simulink model "ADCS_sim"  (R2018b)
settings: Solver=VariableStepAuto  StartTime=0.0  StopTime=T
values from neighbouring files (symbols this model uses):
  A_i = [A_sc(1); A_sc(2); A_sc(3); A_sc(1); A_sc(2); A_sc(3);            A_sa; A_sa; A_sa; A_sa]'    [data_setup.m]
  G = [1 10 1e-4 1e-4 1e-4 1e-4]    [main.m]
  mag_res = [1; 1; 1]*1e-3    [data_setup.m]
  n = length(t)    [main.m]
  n_i = [eye(3), -eye(3), n_sa, -n_sa, n_sa, -n_sa]    [data_setup.m]
  P = zeros(18,18,nF)    [main_test_ekf.m]
  r_i = [CG_1, CG_2, CG_3, CG_4, CG_5, CG_6, CG_7, CG_8, CG_9, CG_10]    [data_setup.m]
  rhoD = ones(1,10)*0.1    [data_setup.m]
  rhoS = [ones(1,6)*0.5, ones(1,4)*0.8]    [data_setup.m]
undefined symbols (not defined in the file or in its folder): A, a, alp_w, Ar, Ar_star, B, C, e, epsilon, fov_star, fov_sun, g1_0, H0, in, Ir, Ixyz, L, mi, n_star_sens, n_sun, n_sun_sens, omega0, omegaE, R_e, R_sun, RAAN, rate_mag, rate_star, rate_sun, sig_mag, sig_star, sig_sun, star_cat, th0
libraries: simulink_extras x9, vrlib x6, dspmathops x5, simulink x5, sharedutil x2, dspmtrx3 x1, dspfactors x1
(part 1 of 2)
settings Model: Creator=Francesco  LastModifiedBy=Francesco
settings DebuggingCC: UnderSpecifiedDimensionMsg=warning

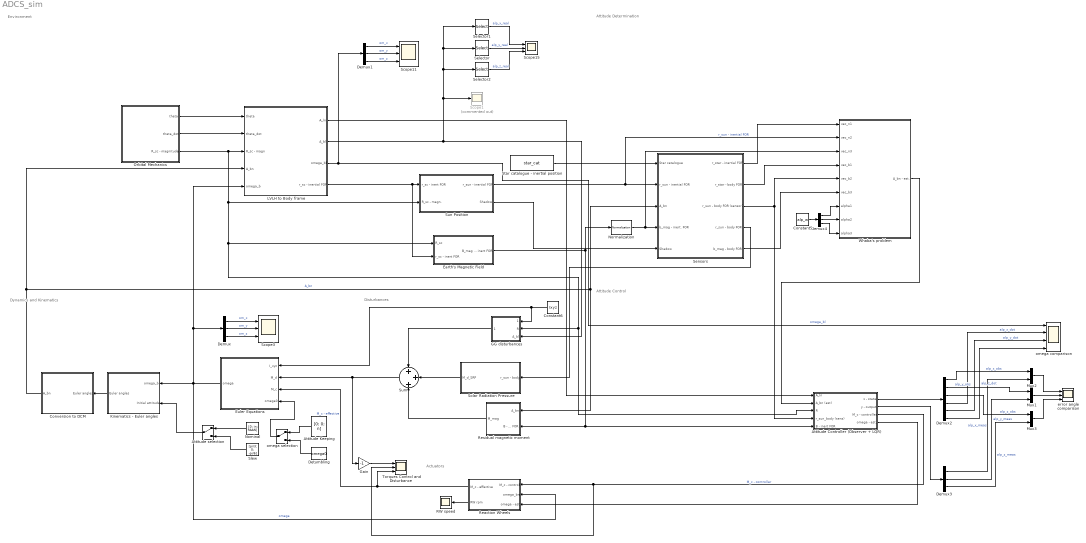
== system ADCS_sim ==
  note: Attitude Control
  note: Dynamics and Kinematics
  note: Attitude Determination
  note: Environment
  note: Actuators
  note: Disturbances
  Attitude Controller (Observer + LQR) : Subsystem
  Attitude Keeping : Constant  Value=[0; 0; n]  VectorParams1D=off
  Attitude selection : ManualSwitch
  Constant5 : Constant  Value=alp_w
  Constant6 : Constant  Value=Ixyz
  Conversion to DCM : Subsystem
  Demux{,1,3..4} (4 alike) : Demux  Outputs=3
  Demux2 : Demux  Outputs=6
  Detumbling : Constant  Value=omega0
  Earth's Magnetic Field : Subsystem
  Euler Equations : Subsystem
  GG disturbances : Subsystem
  Gain : Gain  Gain=-1
  Kinematics - Euler angles : Subsystem
  LVLH to Body frame : Subsystem
  Mux1 : Mux  Inputs=2
  Mux2 : Mux  Inputs=2
  Mux3 : Mux  Inputs=2
  Nominal : Constant  Value=[0; in; RAAN]
  Normalization : dspmathops/Normalization  NormType=2-norm  Bias=1e-10  NormOver=Each column  Dimension=1  roundingMode=Floor  overflowMode=off  accumDataTypeStr=Inherit: Same as product output  accumLastDataTypeStr=Inherit: Same as product output  outputDataTypeStr=Inherit: Same as product output  outputMin=[]  outputMax=[]  outputLastDataTypeStr=Inherit: Same as product output
      settings: SourceProductName=DSP System Toolbox
  Orbital Mechanics : Subsystem
  RW speed : Scope
  Reaction Wheels : Subsystem
  Residual magnetic moment : Subsystem
  Scope1 : Scope  Commented=on
  Scope11 : Scope  NumInputPorts=3
  Scope15 : Scope  NumInputPorts=3
  Scope3 : Scope  NumInputPorts=3
  Selector : Selector  NumberOfDimensions=2  InputPortWidth=3  IndexOptions=Index vector (dialog),Index vector (dialog)  Indices=3,1  OutputSizes=1,1
  Selector1 : Selector  NumberOfDimensions=2  InputPortWidth=3  IndexOptions=Index vector (dialog),Index vector (dialog)  Indices=2,3  OutputSizes=1,1
  Selector2 : Selector  NumberOfDimensions=2  InputPortWidth=3  IndexOptions=Index vector (dialog),Index vector (dialog)  Indices=1,2  OutputSizes=1,1
  Sensors : Subsystem
  Slew : Constant  Value=[pi/3; 0; -pi/6]
  Solar Radiation Pressure : Subsystem  TreatAsAtomicUnit=on
  Star catalogue - inertial position : Constant  Value=star_cat
  Sum : Sum  Inputs=+++
  Sun Position : Subsystem
  Torques Control and Disturbance : Scope  NumInputPorts=3
  Whaba's problem : Subsystem
  error angle comparison : Scope  NumInputPorts=3
  omega comparison : Scope  NumInputPorts=4
  omega selection : ManualSwitch
  wires:
  Demux/2 -> Scope3/2  "om_y"
  LVLH to Body frame/2(A_bl) -> GG disturbances/3(A_bl), Selector/1, Selector1/1, Selector2/1, Scope1/1
  Demux/1 -> Scope3/1  "om_x"
  Demux1/2 -> Scope11/2  "om_y"
  LVLH to Body frame/3(omega_bl) -> omega comparison/1, Demux1/1  "omega_bl"
  Sun Position/1(r_sun - inertial FOR) -> Sensors/2(r_sun - inertial FOR), Whaba's problem/2(vec_n2)  "r_sun - inertial FOR"
  Demux1/1 -> Scope11/1  "om_x"
  Demux/3 -> Scope3/3  "om_z"
  Demux1/3 -> Scope11/3  "om_z"
  Orbital Mechanics/1(theta) -> LVLH to Body frame/1(theta)
  Orbital Mechanics/2(theta_dot) -> LVLH to Body frame/2(theta_dot)
  Euler Equations/1(omega) -> Demux/1, LVLH to Body frame/5(omega_b), Kinematics - Euler angles/1(omega_b), Reaction Wheels/2(omega_bn)  "omega"
  Attitude Keeping/1 -> omega selection/1
  Constant6/1 -> GG disturbances/1("Ix, Iy, Iz"), Euler Equations/1(I_xyz)
  Conversion to DCM/1(A_bn) -> Sensors/3(A_bn), Residual magnetic moment/1(A_bn), LVLH to Body frame/4(A_bn)  "A_bn"
  Residual magnetic moment/1(M_mag) -> Sum/3
  Solar Radiation Pressure/1(M_d_SRP) -> Sum/2
  GG disturbances/1(M_d_GG) -> Sum/1
  Orbital Mechanics/3(R_sc - magnitude) -> LVLH to Body frame/3(R_sc - magn), Attitude Controller (Observer + LQR)/3(R), GG disturbances/2(R), Earth's Magnetic Field/1(R_sc), Sun Position/2(R_sc - magn.)
  LVLH to Body frame/4(r_sc - inertial FOR) -> Earth's Magnetic Field/2(r_sc - inert FOR), Sun Position/1(r_sc - inert FOR)
  Sensors/4(r_sun - body FOR) -> Solar Radiation Pressure/1(r_sun - body)
  Demux2/1 -> Mux2/1  "alp_x_obs"
  Demux2/2 -> Mux1/1  "alp_y_obs"
  Demux3/1 -> Mux2/2  "alp_x_meas"
  Demux3/2 -> Mux1/2  "alp_y_meas"
  Demux2/4 -> omega comparison/2  "alp_x_dot"
  Demux2/5 -> omega comparison/3  "alp_y_dot"
  Demux2/3 -> Mux3/1  "alp_z_obs"
  Demux3/3 -> Mux3/2  "alp_z_meas"
  Demux2/6 -> omega comparison/4  "alp_z_dot"
  Sum/1 -> Euler Equations/2(M_d), Gain/1
  Gain/1 -> Torques Control and Disturbance/1
  Reaction Wheels/1(M_c - effective) -> Euler Equations/3(M_c), Torques Control and Disturbance/3  "M_c - effective"
  Kinematics - Euler angles/1(Euler angles) -> Conversion to DCM/1(Euler angles)
  Star catalogue - inertial position/1 -> Sensors/1(Star catalogue)
  omega selection/1 -> Euler Equations/4(omega0)
  Nominal/1 -> Attitude selection/1
  Attitude selection/1 -> Kinematics - Euler angles/2(Initial attitude)
  Earth's Magnetic Field/1(B_mag - inert FOR) -> Normalization/1, Residual magnetic moment/2(B - inert FOR), Attitude Controller (Observer + LQR)/5(B - inert FOR)
  Constant5/1 -> Demux4/1
  Demux4/1 -> Whaba's problem/7(alpha1)
  Demux4/2 -> Whaba's problem/8(alpha2)
  Demux4/3 -> Whaba's problem/9(alpha3)
  Detumbling/1 -> omega selection/2
  Sun Position/2(Shadow) -> Sensors/5(Shadow)
  Normalization/1 -> Whaba's problem/3(vec_n3), Sensors/4(b_mag - inert. FOR)
  Sensors/5(b_mag - body FOR) -> Whaba's problem/6(vec_b3)
  Sensors/3(r_sun - body FOR (sensor)) -> Attitude Controller (Observer + LQR)/4(r_sun_body (sens)), Whaba's problem/5(vec_b2)
  Sensors/2(r_star - body FOR) -> Whaba's problem/4(vec_b1)
  Selector/1 -> Scope15/2  "alp_y_real"
  Selector1/1 -> Scope15/1  "alp_x_real"
  Selector2/1 -> Scope15/3  "alp_z_real"
  Sensors/1(r_star - inertial FOR) -> Whaba's problem/1(vec_n1)
  Mux2/1 -> error angle comparison/1
  Mux1/1 -> error angle comparison/2
  Mux3/1 -> error angle comparison/3
  Slew/1 -> Attitude selection/2
  Reaction Wheels/2(RW rpm) -> RW speed/1
  Attitude Controller (Observer + LQR)/2(y - output) -> Demux3/1
  Attitude Controller (Observer + LQR)/1(x - state) -> Demux2/1
  Attitude Controller (Observer + LQR)/3(M_c - controller) -> Torques Control and Disturbance/2, Reaction Wheels/1(M_c - control)  "M_c - controller"
  LVLH to Body frame/1(A_ln) -> Attitude Controller (Observer + LQR)/1(A_ln)
  Whaba's problem/1(A_bn - est.) -> Attitude Controller (Observer + LQR)/2(A_bn (est))
  Attitude Controller (Observer + LQR)/4(omega - est.) -> Reaction Wheels/3(omega - est)

== system ADCS_sim/Attitude Controller (Observer + LQR) ==
  A_ln : Inport
  A_bn (est) : Inport  Port=2
  R : Inport  Port=3
  r_sun_body (sens) : Inport  Port=4
  B - inert FOR : Inport  Port=5
  Disturbance Estimator : Subsystem
  "Observer and Controller " : Subsystem
  x - state : Outport
  y - output : Outport  Port=2
  M_c - controller : Outport  Port=3
  omega - est. : Outport  Port=4
  wires:
  "Observer and Controller "/3(M_c - controller) -> M_c - controller/1
  Disturbance Estimator/1(M_d - est.) -> "Observer and Controller "/3(M_d)
  A_ln/1 -> "Observer and Controller "/1(A_ln), Disturbance Estimator/2(A_ln)
  B - inert FOR/1 -> Disturbance Estimator/5(B - inert FOR)
  A_bn (est)/1 -> Disturbance Estimator/4(A_bn), "Observer and Controller "/2(A_bn - est)
  r_sun_body (sens)/1 -> Disturbance Estimator/3(r_sun_body)
  "Observer and Controller "/2(y - output) -> y - output/1
  "Observer and Controller "/1(x - state) -> x - state/1
  "Observer and Controller "/4(omega - est.) -> omega - est./1
  R/1 -> Disturbance Estimator/1(R)

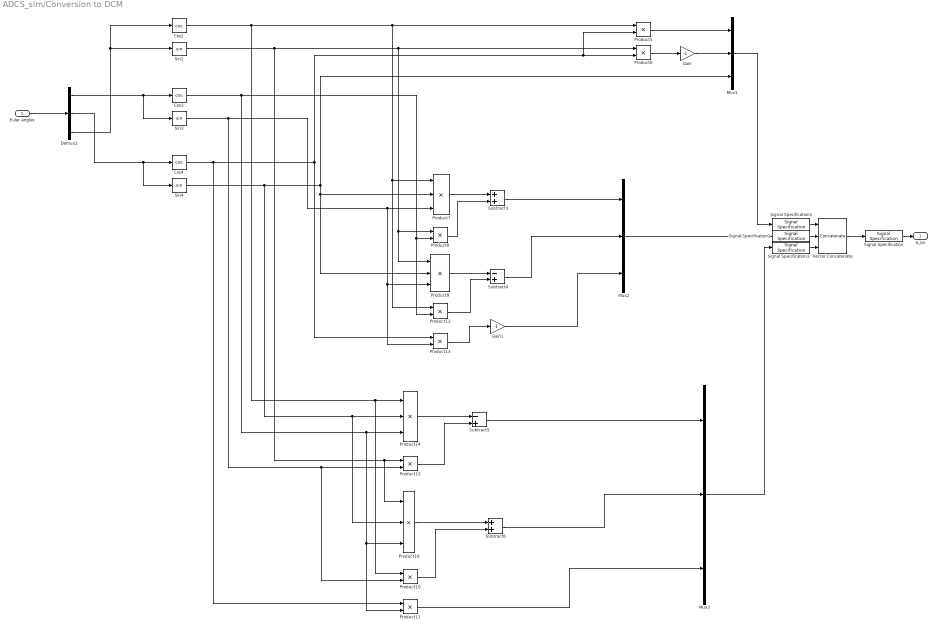
== system ADCS_sim/Conversion to DCM ==
  Euler angles : Inport
  Cos2 : Trigonometry  Operator=cos
  Cos3 : Trigonometry  Operator=cos
  Cos4 : Trigonometry  Operator=cos
  Demux2 : Demux  Outputs=3
  Gain : Gain  Gain=-1
  Gain1 : Gain  Gain=-1
  Mux1 : Mux  Inputs=3
  Mux2 : Mux  Inputs=3
  Mux3 : Mux  Inputs=3
  Product{5..6,8,10..13,15} (8 alike) : Product
  Product{7,9,14,16} (4 alike) : Product  Inputs=3
  Signal Specification : SignalSpecification  Dimensions=[3;3]
  Signal Specification1 : SignalSpecification  Dimensions=[3;1]
  Signal Specification2 : SignalSpecification  Dimensions=[3;1]
  Signal Specification3 : SignalSpecification  Dimensions=[3;1]
  Sin2 : Trigonometry
  Sin3 : Trigonometry
  Sin4 : Trigonometry
  Subtract3 : Sum
  Subtract4 : Sum  Inputs=-+
  Subtract5 : Sum  Inputs=-+
  Subtract6 : Sum
  Vector Concatenate : Concatenate  NumInputs=3  Mode=Multidimensional array  ConcatenateDimension=2
  A_bn : Outport
  wires:
  Product5/1 -> Mux1/1
  Euler angles/1 -> Demux2/1
  Cos2/1 -> Product12/1, Product7/1, Product5/1, Product10/1, Product14/1
  Demux2/3 -> Sin2/1, Cos2/1
  Cos4/1 -> Product11/1, Product13/1, Product5/2, Product6/2
  Subtract5/1 -> Mux3/1
  Mux2/1 -> Signal Specification2/1
  Product15/1 -> Subtract5/2
  Product10/1 -> Subtract6/2
  Sin3/1 -> Product10/2, Product15/2, Product13/2, Product9/3, Product7/3
  Sin2/1 -> Product16/1, Product15/1, Product9/1, Product8/1, Product6/1
  Mux1/1 -> Signal Specification1/1
  Sin4/1 -> Product9/2, Product7/2, Mux1/3, Product16/2, Product14/2
  Product13/1 -> Gain1/1
  Demux2/2 -> Cos4/1, Sin4/1
  Product6/1 -> Gain/1
  Product8/1 -> Subtract3/2
  Product11/1 -> Mux3/3
  Product12/1 -> Subtract4/2
  Demux2/1 -> Sin3/1, Cos3/1
  Cos3/1 -> Product12/2, Product8/2, Product11/2, Product16/3, Product14/3
  Gain1/1 -> Mux2/3
  Product9/1 -> Subtract4/1
  Gain/1 -> Mux1/2
  Subtract3/1 -> Mux2/1
  Subtract6/1 -> Mux3/2
  Product16/1 -> Subtract6/1
  Product14/1 -> Subtract5/1
  Product7/1 -> Subtract3/1
  Subtract4/1 -> Mux2/2
  Vector Concatenate/1 -> Signal Specification/1
  Mux3/1 -> Signal Specification3/1
  Signal Specification/1 -> A_bn/1
  Signal Specification1/1 -> Vector Concatenate/1
  Signal Specification2/1 -> Vector Concatenate/2
  Signal Specification3/1 -> Vector Concatenate/3

== system ADCS_sim/Earth's Magnetic Field ==
  R_sc : Inport
  r_sc - inert FOR : Inport  Port=2
  Constant6 : Constant  Value=H0
  Constant7 : Constant  Value=R_e
  Constant8 : Constant  Value=3
  Divide1 : Product  Inputs=*/
  Dot Product : DotProduct  InputSameDT=on  OutDataTypeStr=Inherit: Inherit via internal rule
  Gain : Gain  Gain=3
  Power : Math  Operator=pow  SaturateOnIntegerOverflow=on
  Product : Product
  Product1 : Product
  Product2 : Product
  Subsystem1 : Subsystem
  Subtract : Sum  Inputs=+-
  B_mag - inert FOR : Outport
  wires:
  Constant7/1 -> Divide1/1
  Power/1 -> Product/2
  Gain/1 -> Product1/2
  Constant6/1 -> Product/1
  r_sc - inert FOR/1 -> Product1/1, Dot Product/1
  Dot Product/1 -> Gain/1
  R_sc/1 -> Divide1/2
  Product/1 -> Product2/1
  Product1/1 -> Subtract/1
  Product2/1 -> B_mag - inert FOR/1
  Subtract/1 -> Product2/2
  Constant8/1 -> Power/2
  Divide1/1 -> Power/1
  Subsystem1/1("m_hat - inert FOR ") -> Dot Product/2, Subtract/2

== system ADCS_sim/Euler Equations ==
  I_xyz : Inport
  M_d : Inport  Port=2
  M_c : Inport  Port=3
  omega0 : Inport  Port=4
  Demux : Demux  Outputs=3
  Demux1 : Demux  Outputs=3
  Divide : Product  Inputs=/*
  Integrator : Integrator  InitialConditionSource=external  InitialCondition=[0.45; 0.52; 0.55]
  Mux : Mux  Inputs=3
  Product : Product  Inputs=3
  Product1 : Product  Inputs=3
  Product2 : Product  Inputs=3
  Subtract : Sum  Inputs=+-
  Subtract1 : Sum  Inputs=+-
  Subtract2 : Sum  Inputs=+-
  Sum : Sum  Inputs=|++
  Sum1 : Sum  Inputs=|++
  omega : Outport
  wires:
  Divide/1 -> Integrator/1  "omega_dot"
  Demux1/1 -> Product2/3, Product1/2
  Demux1/3 -> Product1/3, Product/2
  Subtract1/1 -> Product1/1
  Integrator/1 -> omega/1, Demux1/1  "omega"
  Demux1/2 -> Product2/2, Product/3
  Subtract/1 -> Product/1
  Demux/2 -> Subtract2/2, Subtract/1
  Demux/1 -> Subtract2/1, Subtract1/2
  Demux/3 -> Subtract/2, Subtract1/1
  Mux/1 -> Sum1/1
  omega0/1 -> Integrator/2
  Product1/1 -> Mux/2
  Product/1 -> Mux/1
  Product2/1 -> Mux/3
  Sum/1 -> Sum1/2
  I_xyz/1 -> Divide/1, Demux/1
  Subtract2/1 -> Product2/1
  M_c/1 -> Sum/1
  M_d/1 -> Sum/2
  Sum1/1 -> Divide/2

== system ADCS_sim/GG disturbances ==
  "Ix, Iy, Iz" : Inport
  R : Inport  Port=2
  A_bl : Inport  Port=3
  Constant : Constant  Value=[1; 0; 0]
  Constant1 : Constant  Value=3
  Constant2 : Constant  Value=mi
  Demux2 : Demux  Outputs=3
  Demux3 : Demux  Outputs=3
  Divide : Product  Inputs=*/
  Gain : Gain  Gain=3
  Matrix Multiply2 : Product  Multiplication=Matrix(*)
  Mux : Mux  Inputs=3
  Power : Math  Operator=pow  SaturateOnIntegerOverflow=on
  Product1 : Product  Inputs=4
  Product2 : Product  Inputs=4
  Product3 : Product  Inputs=4
  Subtract1 : Sum  Inputs=+-
  Subtract2 : Sum  Inputs=+-
  Subtract3 : Sum  Inputs=+-
  M_d_GG : Outport
  wires:
  Mux/1 -> M_d_GG/1
  Product2/1 -> Mux/2
  Product3/1 -> Mux/3
  Product1/1 -> Mux/1
  Matrix Multiply2/1 -> Demux3/1
  Subtract3/1 -> Product3/2
  Subtract1/1 -> Product1/2
  Subtract2/1 -> Product2/2
  Demux3/1 -> Product3/3, Product2/3
  "Ix, Iy, Iz"/1 -> Demux2/1
  Demux3/2 -> Product3/4, Product1/4
  Demux2/3 -> Subtract2/2, Subtract1/1
  Constant/1 -> Matrix Multiply2/2
  Demux2/2 -> Subtract3/1, Subtract1/2
  Demux3/3 -> Product2/4, Product1/3
  Demux2/1 -> Subtract3/2, Subtract2/1
  Gain/1 -> Product3/1, Product2/1, Product1/1
  A_bl/1 -> Matrix Multiply2/1
  R/1 -> Power/1
  Constant1/1 -> Power/2
  Divide/1 -> Gain/1
  Power/1 -> Divide/2
  Constant2/1 -> Divide/1

== system ADCS_sim/Kinematics - Euler angles ==
  omega_b : Inport
  Initial attitude : Inport  Port=2
  Cos : Trigonometry  Operator=cos
  Cos1 : Trigonometry  Operator=cos
  Demux : Demux  Outputs=3
  Demux1 : Demux  Outputs=3
  Divide : Product  Inputs=/*
  Integrator : Integrator  InitialConditionSource=external  InitialCondition=[pi/2; pi/2; 0]
  Mux : Mux  Inputs=3
  Product{,1..4} (5 alike) : Product
  Sin : Trigonometry
  Sin1 : Trigonometry
  Subtract : Sum  Inputs=+-
  Subtract1 : Sum
  Subtract2 : Sum  Inputs=-+
  Terminator : Terminator
  Euler angles : Outport
  wires:
  omega_b/1 -> Demux/1
  Demux1/1 -> Terminator/1  "phi"
  Demux1/2 -> Sin/1, Cos/1  "theta"
  Demux1/3 -> Sin1/1, Cos1/1  "psi"
  Demux/1 -> Product3/2, Product/2  "om_u"
  Cos1/1 -> Product2/1, Product/1
  Demux/2 -> Product2/2, Product1/2  "om_v"
  Sin1/1 -> Product3/1, Product1/1
  Product/1 -> Subtract/1
  Product1/1 -> Subtract/2
  Subtract/1 -> Divide/2
  Cos/1 -> Divide/1
  Divide/1 -> Product4/2, Mux/1
  Product2/1 -> Subtract1/1
  Product3/1 -> Subtract1/2
  Subtract1/1 -> Mux/2
  Mux/1 -> Integrator/1  "E.A. dot"
  Demux/3 -> Subtract2/2  "om_w"
  Subtract2/1 -> Mux/3
  Product4/1 -> Subtract2/1
  Sin/1 -> Product4/1
  Integrator/1 -> Demux1/1, Euler angles/1
  Initial attitude/1 -> Integrator/2

== system ADCS_sim/LVLH to Body frame ==
  theta : Inport
  theta_dot : Inport  Port=2
  R_sc - magn : Inport  Port=3
  A_bn : Inport  Port=4
  omega_b : Inport  Port=5
  Constant4 : Constant  Value=in
  Constant7 : Constant  Value=RAAN
  Position vector calculator : Subsystem
  Subsystem1 : Subsystem
  inert2lvlh : Subsystem
  A_ln : Outport
  A_bl : Outport  Port=2
  omega_bl : Outport  Port=3
  r_sc - inertial FOR : Outport  Port=4
  wires:
  Constant4/1 -> inert2lvlh/2(i)
  inert2lvlh/1(A_ln) -> Subsystem1/3(A_ln), A_ln/1  "A_ln"
  theta_dot/1 -> Subsystem1/1(theta_dot)
  Subsystem1/1(A_bl) -> A_bl/1  "A_bl"
  omega_b/1 -> Subsystem1/4(omega_b)
  theta/1 -> Position vector calculator/1(theta), inert2lvlh/1(theta)
  A_bn/1 -> Subsystem1/2(A_bn)
  Subsystem1/2(omega_bl) -> omega_bl/1
  Constant7/1 -> inert2lvlh/3(RAAN)
  Position vector calculator/1(r_n) -> r_sc - inertial FOR/1  "r_sc - inertial FOR"
  inert2lvlh/2(PF 2 ECI) -> Position vector calculator/3(PF 2 ECI)
  R_sc - magn/1 -> Position vector calculator/2(R)

== system ADCS_sim/Orbital Mechanics ==
  Constant : Constant  Value=th0
  Constant1 : Constant  Value=a
  Constant2 : Constant  Value=e
  Constant3 : Constant  Value=mi
  Orbital Mechanics evolut. : Subsystem
  theta : Outport
  theta_dot : Outport  Port=2
  R_sc - magnitude : Outport  Port=3
  wires:
  Constant1/1 -> Orbital Mechanics evolut./2(a)
  Orbital Mechanics evolut./1(theta) -> theta/1
  Orbital Mechanics evolut./3(theta_dot) -> theta_dot/1
  Constant3/1 -> Orbital Mechanics evolut./3(mi)
  Constant2/1 -> Orbital Mechanics evolut./4(e)
  Orbital Mechanics evolut./2(R) -> R_sc - magnitude/1
  Constant/1 -> Orbital Mechanics evolut./1(theta0)

== system ADCS_sim/Reaction Wheels ==
  M_c - control : Inport
  omega_bn : Inport  Port=2
  omega - est : Inport  Port=3
  Reaction Wheels controller : Subsystem
  Reaction Wheels response : Subsystem
  rad/s 2 rpm : Gain  Gain=60/2/pi
  M_c - effective : Outport
  RW rpm : Outport  Port=2
  wires:
  M_c - control/1 -> Reaction Wheels controller/2(M_c - control)
  rad/s 2 rpm/1 -> RW rpm/1  "RW rpm"
  Reaction Wheels controller/1(omega_r) -> rad/s 2 rpm/1, Reaction Wheels response/2(omega_r)
  Reaction Wheels response/1(M_c - effective) -> M_c - effective/1
  omega_bn/1 -> Reaction Wheels response/1(omega_bn)
  omega - est/1 -> Reaction Wheels controller/1(omega_bn)

== system ADCS_sim/Residual magnetic moment ==
  A_bn : Inport
  B - inert FOR : Inport  Port=2
  Constant6 : Constant  Value=mag_res
  Cross Product : vrlib/Utilities/Cross Product
      settings: SourceProductBaseCode=VR
  Matrix Multiply1 : Product  Multiplication=Matrix(*)
  M_mag : Outport
  wires:
  Matrix Multiply1/1 -> Cross Product/2  "b - body FOR"
  B - inert FOR/1 -> Matrix Multiply1/2
  Constant6/1 -> Cross Product/1
  Cross Product/1 -> M_mag/1
  A_bn/1 -> Matrix Multiply1/1

== system ADCS_sim/Sensors ==
  Star catalogue : Inport
  r_sun - inertial FOR : Inport  Port=2
  A_bn : Inport  Port=3
  b_mag - inert. FOR : Inport  Port=4
  Shadow : Inport  Port=5
  Magnetometer error : Subsystem
  Matrix Multiply : Product  Inputs=3  Multiplication=Matrix(*)
  Matrix Multiply1 : Product  Multiplication=Matrix(*)
  Matrix Multiply2 : Product  Multiplication=Matrix(*)
  Product : Product
  Star Sensor error : Subsystem
  Star selector : Subsystem
  Subsystem : Subsystem
  Sun Sensor error : Subsystem
  r_star - inertial FOR : Outport
  r_star - body FOR : Outport  Port=2
  r_sun - body FOR (sensor) : Outport  Port=3
  r_sun - body FOR : Outport  Port=4
  b_mag - body FOR : Outport  Port=5
  wires:
  A_bn/1 -> Matrix Multiply/2, Subsystem/2(A_bn), Star selector/2(A_bn)
  r_sun - inertial FOR/1 -> Product/2
  Star catalogue/1 -> Star selector/1(Star catalogue)
  Star selector/1(r_star - body FOR) -> Matrix Multiply1/2
  Star Sensor error/1(A_eps) -> Matrix Multiply1/1
  Matrix Multiply1/1 -> r_star - body FOR/1
  Star selector/2(r_star - inertial FOR) -> r_star - inertial FOR/1
  Subsystem/1(r_sun - body FOR (sensor)) -> Matrix Multiply2/2
  Sun Sensor error/1(A_eps) -> Matrix Multiply2/1
  Subsystem/2(r_sun -  body FOR) -> r_sun - body FOR/1
  Matrix Multiply2/1 -> r_sun - body FOR (sensor)/1
  b_mag - inert. FOR/1 -> Matrix Multiply/3
  Magnetometer error/1(A_eps) -> Matrix Multiply/1
  Matrix Multiply/1 -> b_mag - body FOR/1
  Shadow/1 -> Product/1
  Product/1 -> Subsystem/1(r_sun - inert FOR)

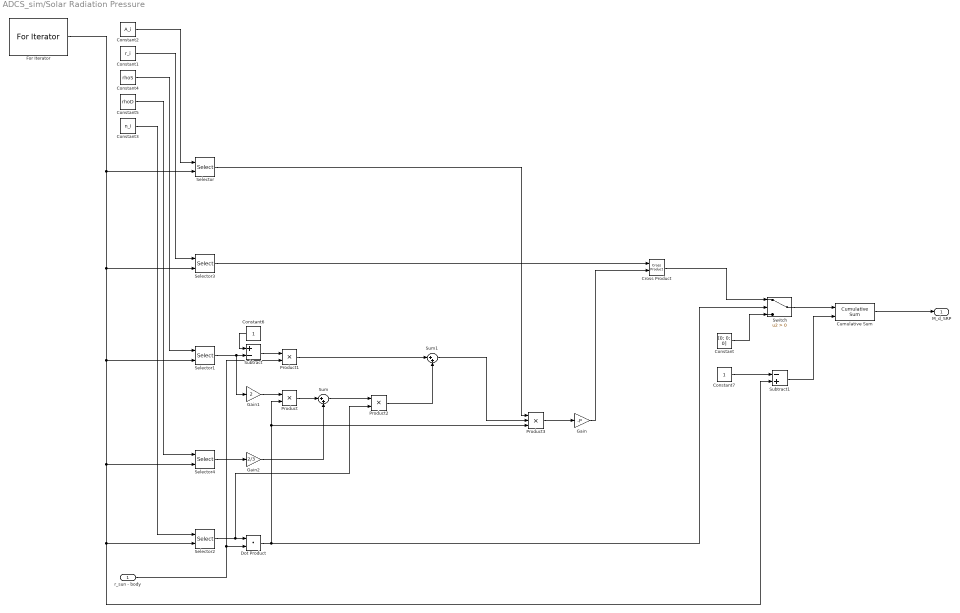
== system ADCS_sim/Solar Radiation Pressure ==
  r_sun - body : Inport
  Constant : Constant  Value=[0; 0; 0]
  Constant1 : Constant  Value=r_i
  Constant2 : Constant  Value=A_i
  Constant3 : Constant  Value=n_i
  Constant4 : Constant  Value=rhoS
  Constant5 : Constant  Value=rhoD
  Constant6 : Constant
  Constant7 : Constant
  Cross Product : vrlib/Utilities/Cross Product
      settings: SourceProductBaseCode=VR
  Cumulative Sum : dspmathops/Cumulative Sum  dim=Channels (running sum)  reset_popup=Falling edge  roundingMode=Floor  overflowMode=off  outputDataTypeStr=Inherit: Same as accumulator  outputMin=[]  outputMax=[]  outputLastDataTypeStr=Inherit: Same as accumulator
      settings: SourceProductName=DSP System Toolbox
  Dot Product : DotProduct  InputSameDT=on  OutDataTypeStr=Inherit: Inherit via internal rule
  For Iterator : ForIterator  IterationLimit=length(A_i)
  Gain : Gain  Gain=-P
  Gain1 : Gain  Gain=2
  Gain2 : Gain  Gain=2/3
  Product : Product
  Product1 : Product
  Product2 : Product
  Product3 : Product  Inputs=3
  Selector{,1..4} (5 alike) : Selector  NumberOfDimensions=2  InputPortWidth=3  IndexOptions=Select all,Index vector (port)  Indices=[1 3],1  OutputSizes=1,1
  Subtract : Sum  Inputs=+-
  Subtract1 : Sum  Inputs=-+
  Sum : Sum  Inputs=|++
  Sum1 : Sum  Inputs=|++
  Switch : Switch  Criteria=u2 > Threshold
  M_d_SRP : Outport
  wires:
  For Iterator/1 -> Selector/2, Selector3/2, Subtract1/2, Selector2/2, Selector4/2, Selector1/2
  Selector/1 -> Product3/1
  Selector3/1 -> Cross Product/1
  Constant3/1 -> Selector2/1
  Selector2/1 -> Product2/2, Dot Product/1
  Constant1/1 -> Selector3/1
  Constant2/1 -> Selector/1
  r_sun - body/1 -> Product1/2, Dot Product/2
  Constant4/1 -> Selector1/1
  Constant5/1 -> Selector4/1
  Selector1/1 -> Subtract/2, Gain1/1
  Constant6/1 -> Subtract/1
  Subtract/1 -> Product1/1
  Dot Product/1 -> Product/2, Product3/3, Switch/2
  Gain1/1 -> Product/1
  Selector4/1 -> Gain2/1
  Product/1 -> Sum/1
  Gain2/1 -> Sum/2
  Sum/1 -> Product2/1
  Product1/1 -> Sum1/1
  Product2/1 -> Sum1/2
  Sum1/1 -> Product3/2
  Product3/1 -> Gain/1
  Gain/1 -> Cross Product/2
  Constant/1 -> Switch/3
  Cross Product/1 -> Switch/1
  Switch/1 -> Cumulative Sum/1
  Subtract1/1 -> Cumulative Sum/2
  Constant7/1 -> Subtract1/1
  Cumulative Sum/1 -> M_d_SRP/1

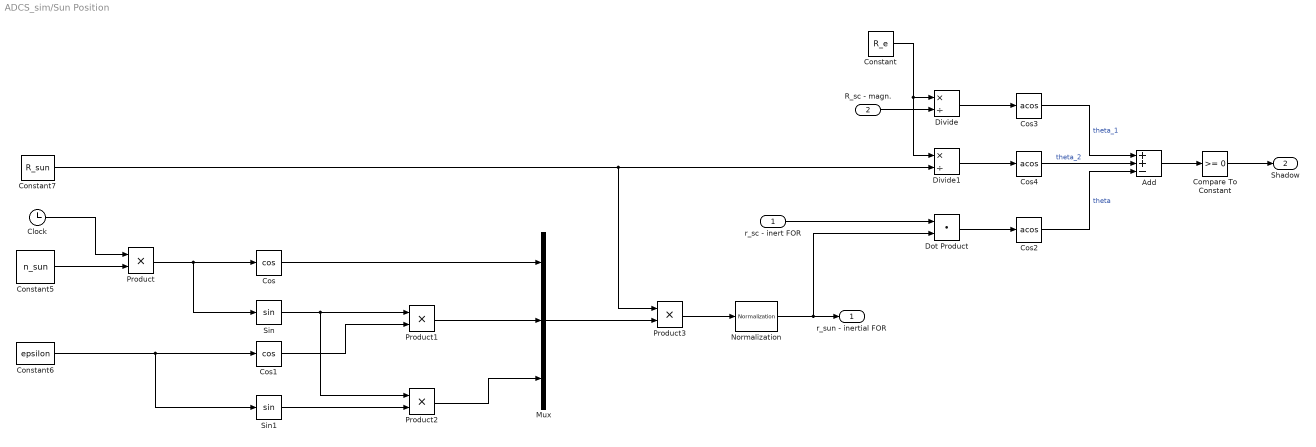
== system ADCS_sim/Sun Position ==
  r_sc - inert FOR : Inport
  R_sc - magn. : Inport  Port=2
  Add : Sum  Inputs=++-
  Clock : Clock
  Compare To Constant : simulink/Logic and Bit Operations/Compare To Constant  relop=>=  const=0  OutDataTypeStr=boolean
  Constant : Constant  Value=R_e
  Constant5 : Constant  Value=n_sun
  Constant6 : Constant  Value=epsilon
  Constant7 : Constant  Value=R_sun
  Cos : Trigonometry  Operator=cos
  Cos1 : Trigonometry  Operator=cos
  Cos2 : Trigonometry  Operator=acos
  Cos3 : Trigonometry  Operator=acos
  Cos4 : Trigonometry  Operator=acos
  Divide : Product  Inputs=*/
  Divide1 : Product  Inputs=*/
  Dot Product : DotProduct  InputSameDT=on  OutDataTypeStr=Inherit: Inherit via internal rule
  Mux : Mux  Inputs=3
  Normalization : dspmathops/Normalization  NormType=2-norm  Bias=1e-10  NormOver=Each column  Dimension=1  roundingMode=Floor  overflowMode=off  accumDataTypeStr=Inherit: Same as product output  accumLastDataTypeStr=Inherit: Same as product output  outputDataTypeStr=Inherit: Same as product output  outputMin=[]  outputMax=[]  outputLastDataTypeStr=Inherit: Same as product output
      settings: SourceProductName=DSP System Toolbox
  Product{,1..3} (4 alike) : Product
  Sin : Trigonometry
  Sin1 : Trigonometry
  r_sun - inertial FOR : Outport
  Shadow : Outport  Port=2
  wires:
  Sin/1 -> Product2/1, Product1/1
  Cos/1 -> Mux/1
  Product/1 -> Sin/1, Cos/1
  Mux/1 -> Product3/2
  Constant6/1 -> Sin1/1, Cos1/1
  Product2/1 -> Mux/3
  Product1/1 -> Mux/2
  Product3/1 -> Normalization/1
  Constant5/1 -> Product/2
  Cos1/1 -> Product1/2
  Clock/1 -> Product/1
  Sin1/1 -> Product2/2
  Constant7/1 -> Product3/1, Divide1/2
  Normalization/1 -> Dot Product/2, r_sun - inertial FOR/1
  r_sc - inert FOR/1 -> Dot Product/1
  Dot Product/1 -> Cos2/1
  Cos2/1 -> Add/3  "theta"
  Constant/1 -> Divide1/1, Divide/1
  R_sc - magn./1 -> Divide/2
  Divide/1 -> Cos3/1
  Divide1/1 -> Cos4/1
  Cos3/1 -> Add/1  "theta_1"
  Cos4/1 -> Add/2  "theta_2"
  Add/1 -> Compare To Constant/1
  Compare To Constant/1 -> Shadow/1

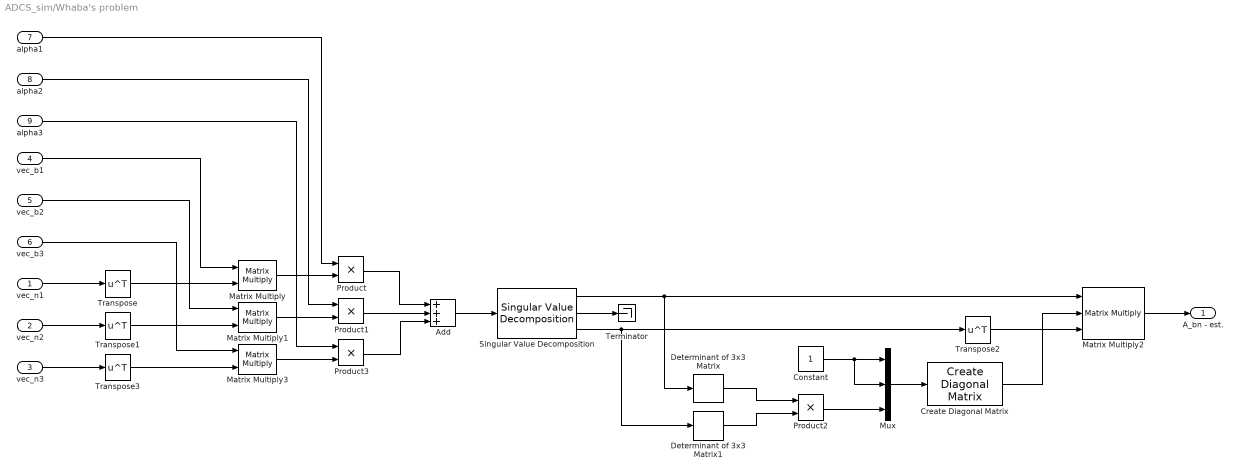
== system ADCS_sim/Whaba's problem ==
  vec_n1 : Inport
  vec_n2 : Inport  Port=2
  vec_n3 : Inport  Port=3
  vec_b1 : Inport  Port=4
  vec_b2 : Inport  Port=5
  vec_b3 : Inport  Port=6
  alpha1 : Inport  Port=7
  alpha2 : Inport  Port=8
  alpha3 : Inport  Port=9
  Add : Sum  Inputs=+++
  Constant : Constant
  Create Diagonal Matrix : dspmtrx3/Create Diagonal Matrix
      settings: SourceProductName=DSP System Toolbox  SourceProductBaseCode=DS
  Determinant of 3x3 Matrix : sharedutil/Determinant of 3x3 Matrix  aMode=aMode
      settings: SourceProductName=Aerospace Blockset  SourceProductBaseCode=AE
  Determinant of 3x3 Matrix1 : sharedutil/Determinant of 3x3 Matrix  aMode=aMode
      settings: SourceProductName=Aerospace Blockset  SourceProductBaseCode=AE
  Matrix Multiply : Product  Multiplication=Matrix(*)
  Matrix Multiply1 : Product  Multiplication=Matrix(*)
  Matrix Multiply2 : Product  Inputs=3  Multiplication=Matrix(*)
  Matrix Multiply3 : Product  Multiplication=Matrix(*)
  Mux : Mux  Inputs=3
  Product{,1..3} (4 alike) : Product
  Singular Value Decomposition : dspfactors/Singular Value Decomposition  wantv=on  wanterr=off  SimulateUsing=Interpreted execution
      settings: SourceProductName=DSP System Toolbox  SourceProductBaseCode=DS
  Terminator : Terminator
  Transpose{,1..3} (4 alike) : Math  Operator=transpose  SaturateOnIntegerOverflow=on
  A_bn - est. : Outport
  wires:
  vec_n1/1 -> Transpose/1
  vec_n2/1 -> Transpose1/1
  Transpose/1 -> Matrix Multiply/2
  vec_b1/1 -> Matrix Multiply/1
  Transpose1/1 -> Matrix Multiply1/2
  vec_b2/1 -> Matrix Multiply1/1
  Matrix Multiply/1 -> Product/2
  Matrix Multiply1/1 -> Product1/2
  alpha2/1 -> Product1/1
  alpha1/1 -> Product/1
  Product/1 -> Add/1
  Product1/1 -> Add/2
  Add/1 -> Singular Value Decomposition/1
  Singular Value Decomposition/2 -> Terminator/1
  Singular Value Decomposition/1 -> Determinant of 3x3 Matrix/1, Matrix Multiply2/1
  Singular Value Decomposition/3 -> Transpose2/1, Determinant of 3x3 Matrix1/1
  Determinant of 3x3 Matrix/1 -> Product2/1
  Determinant of 3x3 Matrix1/1 -> Product2/2
  Product2/1 -> Mux/3
  Constant/1 -> Mux/2, Mux/1
  Mux/1 -> Create Diagonal Matrix/1
  Create Diagonal Matrix/1 -> Matrix Multiply2/2
  Transpose2/1 -> Matrix Multiply2/3
  Matrix Multiply2/1 -> A_bn - est./1
  Product3/1 -> Add/3
  Matrix Multiply3/1 -> Product3/2
  Transpose3/1 -> Matrix Multiply3/2
  vec_n3/1 -> Transpose3/1
  vec_b3/1 -> Matrix Multiply3/1
  alpha3/1 -> Product3/1

== system ADCS_sim/Attitude Controller (Observer + LQR)/Disturbance Estimator ==
  R : Inport
  A_ln : Inport  Port=2
  r_sun_body : Inport  Port=3
  A_bn : Inport  Port=4
  B - inert FOR : Inport  Port=5
  Constant5 : Constant  Value=Ixyz
  GG disturbances1 : Subsystem
  Matrix Multiply2 : Product  Multiplication=Matrix(*)
  Solar Radiation Pressure : Subsystem  TreatAsAtomicUnit=on
  Subsystem3 : Subsystem
  Sum1 : Sum  Inputs=+++
  Transpose : Math  Operator=transpose  SaturateOnIntegerOverflow=on
  M_d - est. : Outport
  wires:
  GG disturbances1/1(M_d_GG) -> Sum1/1
  Constant5/1 -> GG disturbances1/1("Ix, Iy, Iz")
  Subsystem3/1(M_mag) -> Sum1/3
  Solar Radiation Pressure/1(M_d_SRP) -> Sum1/2
  Sum1/1 -> M_d - est./1
  r_sun_body/1 -> Solar Radiation Pressure/1(r_sun - body)
  R/1 -> GG disturbances1/2(R)
  B - inert FOR/1 -> Subsystem3/2(B - inert FOR)
  A_ln/1 -> Transpose/1
  Transpose/1 -> Matrix Multiply2/2
  A_bn/1 -> Subsystem3/1(A_bn), Matrix Multiply2/1
  Matrix Multiply2/1 -> GG disturbances1/3(A_bl)

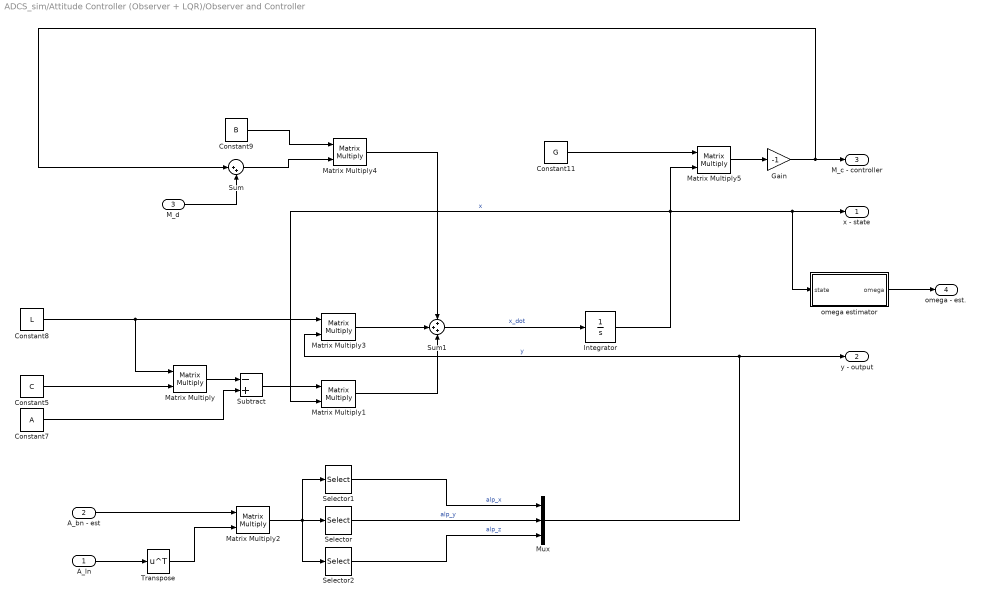
== system ADCS_sim/Attitude Controller (Observer + LQR)/Observer and Controller  ==
  A_ln : Inport
  A_bn - est : Inport  Port=2
  M_d : Inport  Port=3
  Constant11 : Constant  Value=G
  Constant5 : Constant  Value=C
  Constant7 : Constant  Value=A
  Constant8 : Constant  Value=L
  Constant9 : Constant  Value=B
  Gain : Gain  Gain=-1
  Integrator : Integrator  InitialCondition=[0; 0; 0; 0; 0; 0]
  Matrix Multiply{,1..5} (6 alike) : Product  Multiplication=Matrix(*)
  Mux : Mux  Inputs=3
  Selector : Selector  NumberOfDimensions=2  InputPortWidth=3  IndexOptions=Index vector (dialog),Index vector (dialog)  Indices=3,1  OutputSizes=1,1
  Selector1 : Selector  NumberOfDimensions=2  InputPortWidth=3  IndexOptions=Index vector (dialog),Index vector (dialog)  Indices=2,3  OutputSizes=1,1
  Selector2 : Selector  NumberOfDimensions=2  InputPortWidth=3  IndexOptions=Index vector (dialog),Index vector (dialog)  Indices=1,2  OutputSizes=1,1
  Subtract : Sum  Inputs=-+
  Sum : Sum  Inputs=|++
  Sum1 : Sum  Inputs=+++
  Transpose : Math  Operator=transpose  SaturateOnIntegerOverflow=on
  omega estimator : Subsystem
  x - state : Outport
  y - output : Outport  Port=2
  M_c - controller : Outport  Port=3
  omega - est. : Outport  Port=4
  wires:
  Matrix Multiply4/1 -> Sum1/1
  Matrix Multiply2/1 -> Selector2/1, Selector1/1, Selector/1
  Constant9/1 -> Matrix Multiply4/1
  Integrator/1 -> Matrix Multiply1/2, Matrix Multiply5/2, omega estimator/1(state), x - state/1  "x"
  Matrix Multiply5/1 -> Gain/1
  Selector2/1 -> Mux/3  "alp_z"
  Matrix Multiply3/1 -> Sum1/2
  Selector1/1 -> Mux/1  "alp_x"
  Constant5/1 -> Matrix Multiply/2
  Mux/1 -> y - output/1, Matrix Multiply3/2  "y"
  Constant8/1 -> Matrix Multiply/1, Matrix Multiply3/1
  Selector/1 -> Mux/2  "alp_y"
  Matrix Multiply/1 -> Subtract/1
  Matrix Multiply1/1 -> Sum1/3
  Transpose/1 -> Matrix Multiply2/2
  Subtract/1 -> Matrix Multiply1/1
  A_ln/1 -> Transpose/1
  Constant11/1 -> Matrix Multiply5/1
  Sum1/1 -> Integrator/1  "x_dot"
  M_d/1 -> Sum/2
  Constant7/1 -> Subtract/2
  A_bn - est/1 -> Matrix Multiply2/1
  Gain/1 -> Sum/1, M_c - controller/1
  Sum/1 -> Matrix Multiply4/2
  omega estimator/1(omega) -> omega - est./1

== system ADCS_sim/Earth's Magnetic Field/Subsystem1 ==
  Clock : Clock
  Constant6 : Constant  Value=omegaE
  Constant7 : Constant  Value=acos(g1_0/H0)  VectorParams1D=off
  Cos : Trigonometry  Operator=cos
  Cos1 : Trigonometry  Operator=cos
  Mux : Mux  Inputs=3
  Product : Product
  Product1 : Product
  Product2 : Product
  Sin : Trigonometry
  Sin1 : Trigonometry
  "m_hat - inert FOR " : Outport
  wires:
  Cos/1 -> Mux/3
  Sin/1 -> Product2/1, Product1/1
  Mux/1 -> "m_hat - inert FOR "/1
  Clock/1 -> Product/2
  Cos1/1 -> Product1/2
  Product/1 -> Cos1/1, Sin1/1
  Constant6/1 -> Product/1
  Product2/1 -> Mux/2
  Constant7/1 -> Sin/1, Cos/1
  Product1/1 -> Mux/1
  Sin1/1 -> Product2/2

== system ADCS_sim/LVLH to Body frame/Position vector calculator ==
  theta : Inport
  R : Inport  Port=2
  PF 2 ECI : Inport  Port=3
  Constant : Constant  Value=0
  Cos : Trigonometry  Operator=cos
  Matrix Multiply : Product  Multiplication=Matrix(*)
  Mux : Mux  Inputs=3
  Normalization : dspmathops/Normalization  NormType=2-norm  Bias=1e-10  NormOver=Each column  Dimension=1  roundingMode=Floor  overflowMode=off  accumDataTypeStr=Inherit: Same as product output  accumLastDataTypeStr=Inherit: Same as product output  outputDataTypeStr=Inherit: Same as product output  outputMin=[]  outputMax=[]  outputLastDataTypeStr=Inherit: Same as product output
      settings: SourceProductName=DSP System Toolbox
  Product2 : Product
  Sin : Trigonometry
  r_n : Outport
  wires:
  theta/1 -> Sin/1, Cos/1
  Sin/1 -> Mux/2
  Mux/1 -> Product2/2
  Constant/1 -> Mux/3
  Cos/1 -> Mux/1
  R/1 -> Product2/1
  Product2/1 -> Normalization/1
  Normalization/1 -> Matrix Multiply/2
  Matrix Multiply/1 -> r_n/1
  PF 2 ECI/1 -> Matrix Multiply/1

== system ADCS_sim/LVLH to Body frame/Subsystem1 ==
  theta_dot : Inport
  A_bn : Inport  Port=2
  A_ln : Inport  Port=3
  omega_b : Inport  Port=4
  Constant5 : Constant  Value=0
  Matrix Multiply : Product  Multiplication=Matrix(*)
  Matrix Multiply1 : Product  Multiplication=Matrix(*)
  Mux : Mux  Inputs=3
  Subtract : Sum  Inputs=+-
  Transpose : Math  Operator=transpose  SaturateOnIntegerOverflow=on
  A_bl : Outport
  omega_bl : Outport  Port=2
  wires:
  A_bn/1 -> Matrix Multiply/1
  omega_b/1 -> Subtract/1
  Matrix Multiply/1 -> Matrix Multiply1/1, A_bl/1  "A_bl"
  Matrix Multiply1/1 -> Subtract/2  "omega"
  Mux/1 -> Matrix Multiply1/2
  A_ln/1 -> Transpose/1
  Constant5/1 -> Mux/2, Mux/1
  Transpose/1 -> Matrix Multiply/2
  theta_dot/1 -> Mux/3
  Subtract/1 -> omega_bl/1

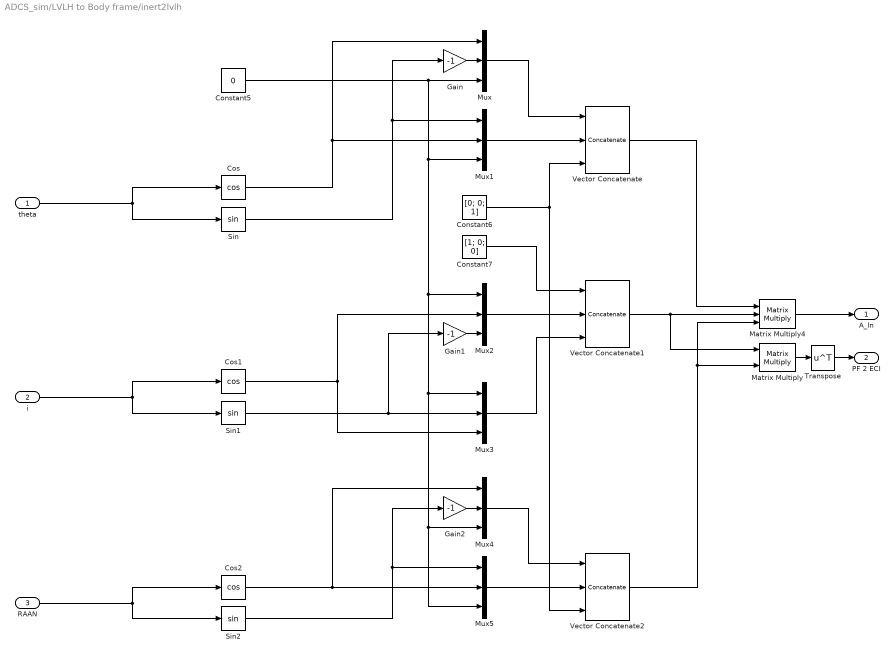
== system ADCS_sim/LVLH to Body frame/inert2lvlh ==
  theta : Inport
  i : Inport  Port=2
  RAAN : Inport  Port=3
  Constant5 : Constant  Value=0
  Constant6 : Constant  Value=[0; 0; 1]
  Constant7 : Constant  Value=[1; 0; 0]
  Cos : Trigonometry  Operator=cos
  Cos1 : Trigonometry  Operator=cos
  Cos2 : Trigonometry  Operator=cos
  Gain : Gain  Gain=-1
  Gain1 : Gain  Gain=-1
  Gain2 : Gain  Gain=-1
  Matrix Multiply : Product  Multiplication=Matrix(*)
  Matrix Multiply4 : Product  Inputs=3  Multiplication=Matrix(*)
  Mux{,1..5} (6 alike) : Mux  Inputs=3
  Sin : Trigonometry
  Sin1 : Trigonometry
  Sin2 : Trigonometry
  Transpose : Math  Operator=transpose  SaturateOnIntegerOverflow=on
  Vector Concatenate : Concatenate  NumInputs=3  Mode=Multidimensional array  ConcatenateDimension=2
  Vector Concatenate1 : Concatenate  NumInputs=3  Mode=Multidimensional array  ConcatenateDimension=2
  Vector Concatenate2 : Concatenate  NumInputs=3  Mode=Multidimensional array  ConcatenateDimension=2
  A_ln : Outport
  PF 2 ECI : Outport  Port=2
  wires:
  Cos/1 -> Mux1/2, Mux/1
  i/1 -> Sin1/1, Cos1/1
  Mux3/1 -> Vector Concatenate1/3
  Constant7/1 -> Vector Concatenate1/1
  Constant5/1 -> Mux3/1, Mux5/3, Mux4/3, Mux2/1, Mux1/3, Mux/3
  Gain1/1 -> Mux2/3
  Vector Concatenate/1 -> Matrix Multiply4/1
  Sin/1 -> Gain/1, Mux1/1
  Mux2/1 -> Vector Concatenate1/2
  Gain/1 -> Mux/2
  Sin1/1 -> Gain1/1, Mux3/2
  Constant6/1 -> Vector Concatenate/3, Vector Concatenate2/3
  Matrix Multiply4/1 -> A_ln/1
  Mux1/1 -> Vector Concatenate/2
  theta/1 -> Sin/1, Cos/1
  Vector Concatenate1/1 -> Matrix Multiply/1, Matrix Multiply4/2
  Mux/1 -> Vector Concatenate/1
  Cos1/1 -> Mux2/2, Mux3/3
  Gain2/1 -> Mux4/2
  Mux4/1 -> Vector Concatenate2/1
  Sin2/1 -> Gain2/1, Mux5/1
  Mux5/1 -> Vector Concatenate2/2
  Vector Concatenate2/1 -> Matrix Multiply/2, Matrix Multiply4/3
  Cos2/1 -> Mux5/2, Mux4/1
  RAAN/1 -> Sin2/1, Cos2/1
  Matrix Multiply/1 -> Transpose/1
  Transpose/1 -> PF 2 ECI/1

== system ADCS_sim/Orbital Mechanics/Orbital Mechanics evolut. ==
  theta0 : Inport
  a : Inport  Port=2
  mi : Inport  Port=3
  e : Inport  Port=4
  Integrator : Integrator  InitialConditionSource=external
  Radius : Subsystem
  True An. evolut. : Subsystem
  theta : Outport
  R : Outport  Port=2
  theta_dot : Outport  Port=3
  wires:
  Radius/1(R) -> R/1
  theta0/1 -> Integrator/2
  e/1 -> Radius/3(e), True An. evolut./2(e)
  a/1 -> Radius/2(a), True An. evolut./1(a)
  True An. evolut./1(theta_dot) -> theta_dot/1, Integrator/1
  Integrator/1 -> theta/1, Radius/1(theta), True An. evolut./4(" theta ")
  mi/1 -> True An. evolut./3(mi)

== system ADCS_sim/Reaction Wheels/Reaction Wheels controller ==
  omega_bn : Inport
  M_c - control : Inport  Port=2
  Constant7 : Constant  Value=Ar_star
  Constant8 : Constant  Value=Ar
  Constant9 : Constant  Value=Ir
  Cross Product1 : vrlib/Utilities/Cross Product
      settings: SourceProductBaseCode=VR
  Divide : Product  Inputs=*/
  Gain : Gain  Gain=-1
  Integrator : Integrator  InitialCondition=[0; 0; 0; 0]
  Matrix Multiply6 : Product  Multiplication=Matrix(*)
  Matrix Multiply7 : Product  Multiplication=Matrix(*)
  Product : Product
  Saturation : Saturate  UpperLimit=628.32  LowerLimit=-628.32
  Saturation1 : Saturate  UpperLimit=1e-3  LowerLimit=-1e-3
  Subtract : Sum
  omega_r : Outport
  wires:
  Matrix Multiply7/1 -> Gain/1  "hr_dot"
  Integrator/1 -> Saturation/1  "omega_r"
  Matrix Multiply6/1 -> Cross Product1/2
  Constant9/1 -> Divide/2, Product/2
  Cross Product1/1 -> Subtract/2
  Divide/1 -> Integrator/1  "omega_r_dot"
  Constant8/1 -> Matrix Multiply6/1
  omega_bn/1 -> Cross Product1/1
  Subtract/1 -> Matrix Multiply7/2
  Product/1 -> Matrix Multiply6/2
  M_c - control/1 -> Subtract/1
  Gain/1 -> Saturation1/1
  Constant7/1 -> Matrix Multiply7/1
  Saturation/1 -> Product/1, omega_r/1
  Saturation1/1 -> Divide/1

== system ADCS_sim/Reaction Wheels/Reaction Wheels response ==
  omega_bn : Inport
  omega_r : Inport  Port=2
  Constant7 : Constant  Value=Ar
  Constant8 : Constant  Value=Ir
  Cross Product1 : vrlib/Utilities/Cross Product
      settings: SourceProductBaseCode=VR
  Derivative : Derivative
  Gain : Gain  Gain=-1
  Matrix Multiply6 : Product  Multiplication=Matrix(*)
  Matrix Multiply7 : Product  Multiplication=Matrix(*)
  Product : Product
  Product1 : Product
  Subtract : Sum  Inputs=+-
  M_c - effective : Outport
  wires:
  Matrix Multiply6/1 -> Cross Product1/2
  Subtract/1 -> M_c - effective/1
  Constant7/1 -> Matrix Multiply7/1, Matrix Multiply6/1
  Cross Product1/1 -> Subtract/1
  omega_bn/1 -> Gain/1
  Product/1 -> Matrix Multiply6/2
  Constant8/1 -> Product1/1, Product/2
  Gain/1 -> Cross Product1/1
  omega_r/1 -> Derivative/1, Product/1
  Matrix Multiply7/1 -> Subtract/2
  Derivative/1 -> Product1/2
  Product1/1 -> Matrix Multiply7/2

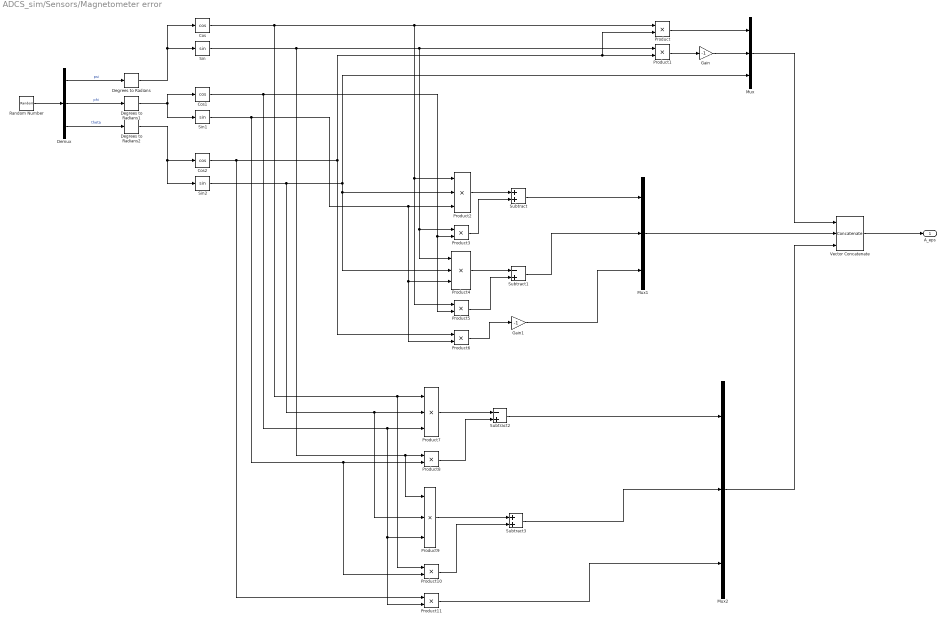
== system ADCS_sim/Sensors/Magnetometer error ==
  Cos : Trigonometry  Operator=cos
  Cos1 : Trigonometry  Operator=cos
  Cos2 : Trigonometry  Operator=cos
  Degrees to Radians : simulink_extras/Transformations/Degrees to Radians
  Degrees to Radians1 : simulink_extras/Transformations/Degrees to Radians
  Degrees to Radians2 : simulink_extras/Transformations/Degrees to Radians
  Demux : Demux  Outputs=3
  Gain : Gain  Gain=-1
  Gain1 : Gain  Gain=-1
  Mux : Mux  Inputs=3
  Mux1 : Mux  Inputs=3
  Mux2 : Mux  Inputs=3
  Product{,1,3,5..6,8,10..11} (8 alike) : Product
  Product{2,4,7,9} (4 alike) : Product  Inputs=3
  Random Number : RandomNumber  Variance=sig_mag^2  Seed=[10;11;12]  SampleTime=1/rate_mag
  Sin : Trigonometry
  Sin1 : Trigonometry
  Sin2 : Trigonometry
  Subtract : Sum
  Subtract1 : Sum  Inputs=-+
  Subtract2 : Sum  Inputs=-+
  Subtract3 : Sum
  Vector Concatenate : Concatenate  NumInputs=3  Mode=Multidimensional array  ConcatenateDimension=2
  A_eps : Outport
  wires:
  Product5/1 -> Subtract1/2
  Sin1/1 -> Product10/2, Product8/2, Product6/2, Product4/3, Product2/3
  Gain/1 -> Mux/2
  Cos1/1 -> Product5/2, Product3/2, Product11/2, Product9/3, Product7/3
  Gain1/1 -> Mux1/3
  Cos/1 -> Product5/1, Product2/1, Product/1, Product10/1, Product7/1
  Cos2/1 -> Product11/1, Product6/1, Product/2, Product1/2
  Product11/1 -> Mux2/3
  Sin2/1 -> Product4/2, Product2/2, Mux/3, Product9/2, Product7/2
  Product4/1 -> Subtract1/1
  Demux/3 -> Degrees to Radians2/1  "theta"
  Mux/1 -> Vector Concatenate/1
  Product/1 -> Mux/1
  Demux/2 -> Degrees to Radians1/1  "phi"
  Product8/1 -> Subtract2/2
  Sin/1 -> Product9/1, Product8/1, Product4/1, Product3/1, Product1/1
  Vector Concatenate/1 -> A_eps/1
  Degrees to Radians2/1 -> Cos2/1, Sin2/1
  Mux1/1 -> Vector Concatenate/2
  Subtract2/1 -> Mux2/1
  Subtract3/1 -> Mux2/2
  Mux2/1 -> Vector Concatenate/3
  Product6/1 -> Gain1/1
  Degrees to Radians/1 -> Sin/1, Cos/1
  Product7/1 -> Subtract2/1
  Demux/1 -> Degrees to Radians/1  "psi"
  Degrees to Radians1/1 -> Sin1/1, Cos1/1
  Subtract1/1 -> Mux1/2
  Product10/1 -> Subtract3/2
  Product2/1 -> Subtract/1
  Product3/1 -> Subtract/2
  Subtract/1 -> Mux1/1
  Product1/1 -> Gain/1
  Product9/1 -> Subtract3/1
  Random Number/1 -> Demux/1

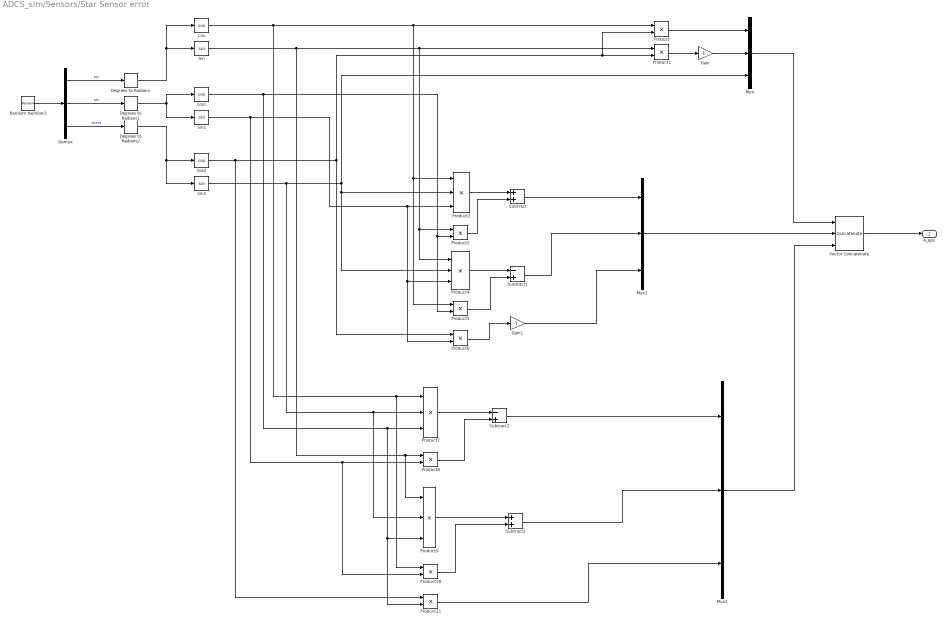
== system ADCS_sim/Sensors/Star Sensor error ==
  Cos : Trigonometry  Operator=cos
  Cos1 : Trigonometry  Operator=cos
  Cos2 : Trigonometry  Operator=cos
  Degrees to Radians : simulink_extras/Transformations/Degrees to Radians
  Degrees to Radians1 : simulink_extras/Transformations/Degrees to Radians
  Degrees to Radians2 : simulink_extras/Transformations/Degrees to Radians
  Demux : Demux  Outputs=3
  Gain : Gain  Gain=-1
  Gain1 : Gain  Gain=-1
  Mux : Mux  Inputs=3
  Mux1 : Mux  Inputs=3
  Mux2 : Mux  Inputs=3
  Product{,1,3,5..6,8,10..11} (8 alike) : Product
  Product{2,4,7,9} (4 alike) : Product  Inputs=3
  Random Number3 : RandomNumber  Variance=sig_star^2  Seed=[4; 5; 6]  SampleTime=1/rate_star
  Sin : Trigonometry
  Sin1 : Trigonometry
  Sin2 : Trigonometry
  Subtract : Sum
  Subtract1 : Sum  Inputs=-+
  Subtract2 : Sum  Inputs=-+
  Subtract3 : Sum
  Vector Concatenate : Concatenate  NumInputs=3  Mode=Multidimensional array  ConcatenateDimension=2
  A_eps : Outport
  wires:
  Product5/1 -> Subtract1/2
  Sin1/1 -> Product10/2, Product8/2, Product6/2, Product4/3, Product2/3
  Gain/1 -> Mux/2
  Cos1/1 -> Product5/2, Product3/2, Product11/2, Product9/3, Product7/3
  Gain1/1 -> Mux1/3
  Cos/1 -> Product5/1, Product2/1, Product/1, Product10/1, Product7/1
  Cos2/1 -> Product11/1, Product6/1, Product/2, Product1/2
  Product11/1 -> Mux2/3
  Sin2/1 -> Product4/2, Product2/2, Mux/3, Product9/2, Product7/2
  Product4/1 -> Subtract1/1
  Mux/1 -> Vector Concatenate/1
  Product/1 -> Mux/1
  Product8/1 -> Subtract2/2
  Sin/1 -> Product9/1, Product8/1, Product4/1, Product3/1, Product1/1
  Vector Concatenate/1 -> A_eps/1
  Degrees to Radians2/1 -> Cos2/1, Sin2/1
  Mux1/1 -> Vector Concatenate/2
  Subtract2/1 -> Mux2/1
  Subtract3/1 -> Mux2/2
  Mux2/1 -> Vector Concatenate/3
  Product6/1 -> Gain1/1
  Degrees to Radians/1 -> Sin/1, Cos/1
  Product7/1 -> Subtract2/1
  Degrees to Radians1/1 -> Sin1/1, Cos1/1
  Subtract1/1 -> Mux1/2
  Product10/1 -> Subtract3/2
  Product2/1 -> Subtract/1
  Product3/1 -> Subtract/2
  Subtract/1 -> Mux1/1
  Product1/1 -> Gain/1
  Product9/1 -> Subtract3/1
  Demux/2 -> Degrees to Radians1/1  "phi"
  Demux/3 -> Degrees to Radians2/1  "theta"
  Random Number3/1 -> Demux/1
  Demux/1 -> Degrees to Radians/1  "psi"

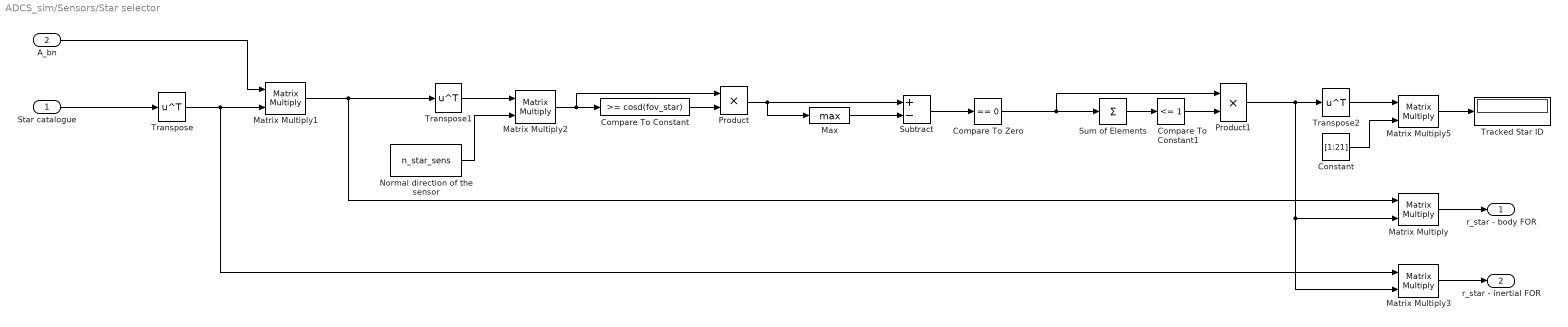
== system ADCS_sim/Sensors/Star selector ==
  Star catalogue : Inport
  A_bn : Inport  Port=2
  Compare To Constant : simulink/Logic and Bit Operations/Compare To Constant  relop=>=  const=cosd(fov_star)  OutDataTypeStr=boolean
  Compare To Constant1 : simulink/Logic and Bit Operations/Compare To Constant  relop=<=  const=1  OutDataTypeStr=boolean
  Compare To Zero : simulink/Logic and Bit Operations/Compare To Zero  relop===  OutDataTypeStr=boolean
  Constant : Constant  Value=[1:21]
  Matrix Multiply{,1..3,5} (5 alike) : Product  Multiplication=Matrix(*)
  Max : MinMax  Function=max
  Normal direction of the sensor : Constant  Value=n_star_sens
  Product : Product
  Product1 : Product
  Subtract : Sum  Inputs=+-
  Sum of Elements : Sum  Inputs=+
  Tracked Star ID : Display
  Transpose : Math  Operator=transpose  SaturateOnIntegerOverflow=on
  Transpose1 : Math  Operator=transpose  SaturateOnIntegerOverflow=on
  Transpose2 : Math  Operator=transpose  SaturateOnIntegerOverflow=on
  r_star - body FOR : Outport
  r_star - inertial FOR : Outport  Port=2
  wires:
  Matrix Multiply1/1 -> Matrix Multiply/1, Transpose1/1
  Transpose1/1 -> Matrix Multiply2/1
  Star catalogue/1 -> Transpose/1
  Matrix Multiply2/1 -> Compare To Constant/1, Product/1
  Compare To Zero/1 -> Product1/1, Sum of Elements/1
  Max/1 -> Subtract/2
  Transpose/1 -> Matrix Multiply3/1, Matrix Multiply1/2
  A_bn/1 -> Matrix Multiply1/1
  Subtract/1 -> Compare To Zero/1
  Normal direction of the sensor/1 -> Matrix Multiply2/2
  Matrix Multiply3/1 -> r_star - inertial FOR/1
  Matrix Multiply/1 -> r_star - body FOR/1
  Matrix Multiply5/1 -> Tracked Star ID/1
  Constant/1 -> Matrix Multiply5/2
  Transpose2/1 -> Matrix Multiply5/1
  Product/1 -> Max/1, Subtract/1
  Compare To Constant/1 -> Product/2
  Sum of Elements/1 -> Compare To Constant1/1
  Compare To Constant1/1 -> Product1/2
  Product1/1 -> Matrix Multiply3/2, Matrix Multiply/2, Transpose2/1

== system ADCS_sim/Sensors/Subsystem ==
  r_sun - inert FOR : Inport
  A_bn : Inport  Port=2
  Compare To Constant : simulink/Logic and Bit Operations/Compare To Constant  relop=>=  const=cosd(fov_sun)  OutDataTypeStr=boolean
  Constant : Constant  Value=n_sun_sens
  Constant1 : Constant  Value=[0; 0; 0]
  Matrix Multiply : Product  Multiplication=Matrix(*)
  Matrix Multiply1 : Product  Multiplication=Matrix(*)
  Sum of Elements : Sum  Inputs=+
  Switch : Switch  Criteria=u2 > Threshold
  Transpose : Math  Operator=transpose  SaturateOnIntegerOverflow=on
  r_sun - body FOR (sensor) : Outport
  r_sun -  body FOR : Outport  Port=2
  wires:
  A_bn/1 -> Matrix Multiply/1
  r_sun - inert FOR/1 -> Matrix Multiply/2
  Matrix Multiply/1 -> r_sun -  body FOR/1, Switch/1, Matrix Multiply1/2
  Constant/1 -> Transpose/1
  Transpose/1 -> Matrix Multiply1/1
  Matrix Multiply1/1 -> Compare To Constant/1
  Compare To Constant/1 -> Sum of Elements/1
  Sum of Elements/1 -> Switch/2
  Constant1/1 -> Switch/3
  Switch/1 -> r_sun - body FOR (sensor)/1

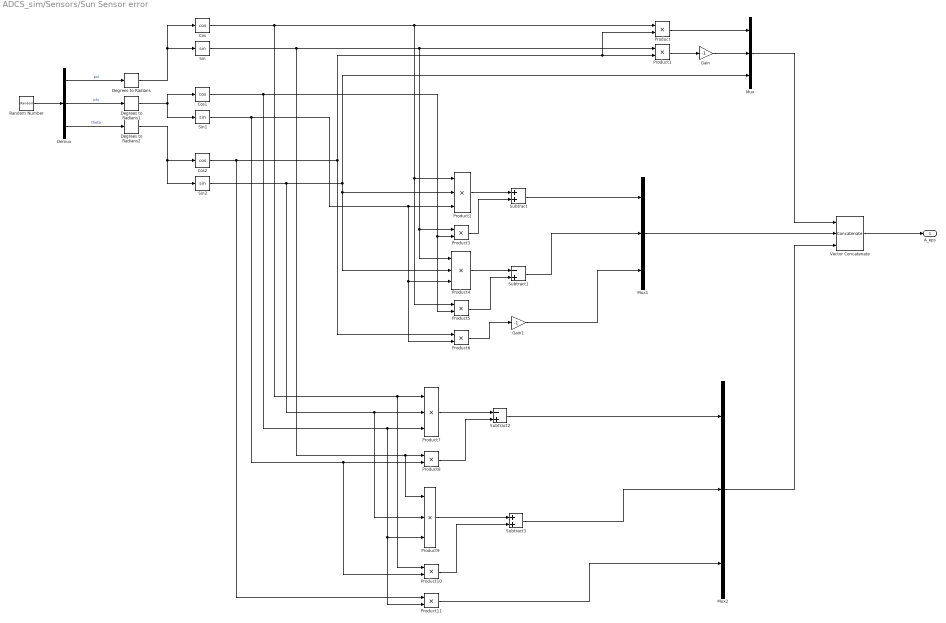
== system ADCS_sim/Sensors/Sun Sensor error ==
  Cos : Trigonometry  Operator=cos
  Cos1 : Trigonometry  Operator=cos
  Cos2 : Trigonometry  Operator=cos
  Degrees to Radians : simulink_extras/Transformations/Degrees to Radians
  Degrees to Radians1 : simulink_extras/Transformations/Degrees to Radians
  Degrees to Radians2 : simulink_extras/Transformations/Degrees to Radians
  Demux : Demux  Outputs=3
  Gain : Gain  Gain=-1
  Gain1 : Gain  Gain=-1
  Mux : Mux  Inputs=3
  Mux1 : Mux  Inputs=3
  Mux2 : Mux  Inputs=3
  Product{,1,3,5..6,8,10..11} (8 alike) : Product
  Product{2,4,7,9} (4 alike) : Product  Inputs=3
  Random Number : RandomNumber  Variance=sig_sun^2  Seed=[1;2;3]  SampleTime=1/rate_sun
  Sin : Trigonometry
  Sin1 : Trigonometry
  Sin2 : Trigonometry
  Subtract : Sum
  Subtract1 : Sum  Inputs=-+
  Subtract2 : Sum  Inputs=-+
  Subtract3 : Sum
  Vector Concatenate : Concatenate  NumInputs=3  Mode=Multidimensional array  ConcatenateDimension=2
  A_eps : Outport
  wires:
  Product5/1 -> Subtract1/2
  Sin1/1 -> Product10/2, Product8/2, Product6/2, Product4/3, Product2/3
  Gain/1 -> Mux/2
  Cos1/1 -> Product5/2, Product3/2, Product11/2, Product9/3, Product7/3
  Gain1/1 -> Mux1/3
  Cos/1 -> Product5/1, Product2/1, Product/1, Product10/1, Product7/1
  Cos2/1 -> Product11/1, Product6/1, Product/2, Product1/2
  Product11/1 -> Mux2/3
  Sin2/1 -> Product4/2, Product2/2, Mux/3, Product9/2, Product7/2
  Product4/1 -> Subtract1/1
  Demux/3 -> Degrees to Radians2/1  "theta"
  Mux/1 -> Vector Concatenate/1
  Product/1 -> Mux/1
  Demux/2 -> Degrees to Radians1/1  "phi"
  Product8/1 -> Subtract2/2
  Sin/1 -> Product9/1, Product8/1, Product4/1, Product3/1, Product1/1
  Vector Concatenate/1 -> A_eps/1
  Degrees to Radians2/1 -> Cos2/1, Sin2/1
  Mux1/1 -> Vector Concatenate/2
  Subtract2/1 -> Mux2/1
  Subtract3/1 -> Mux2/2
  Mux2/1 -> Vector Concatenate/3
  Product6/1 -> Gain1/1
  Degrees to Radians/1 -> Sin/1, Cos/1
  Product7/1 -> Subtract2/1
  Demux/1 -> Degrees to Radians/1  "psi"
  Degrees to Radians1/1 -> Sin1/1, Cos1/1
  Subtract1/1 -> Mux1/2
  Product10/1 -> Subtract3/2
  Product2/1 -> Subtract/1
  Product3/1 -> Subtract/2
  Subtract/1 -> Mux1/1
  Product1/1 -> Gain/1
  Product9/1 -> Subtract3/1
  Random Number/1 -> Demux/1

== system ADCS_sim/Attitude Controller (Observer + LQR)/Disturbance Estimator/GG disturbances1 ==
  "Ix, Iy, Iz" : Inport
  R : Inport  Port=2
  A_bl : Inport  Port=3
  Constant : Constant  Value=[1; 0; 0]
  Constant1 : Constant  Value=3
  Constant2 : Constant  Value=mi
  Demux2 : Demux  Outputs=3
  Demux3 : Demux  Outputs=3
  Divide : Product  Inputs=*/
  Gain : Gain  Gain=3
  Matrix Multiply2 : Product  Multiplication=Matrix(*)
  Mux : Mux  Inputs=3
  Power : Math  Operator=pow  SaturateOnIntegerOverflow=on
  Product1 : Product  Inputs=4
  Product2 : Product  Inputs=4
  Product3 : Product  Inputs=4
  Subtract1 : Sum  Inputs=+-
  Subtract2 : Sum  Inputs=+-
  Subtract3 : Sum  Inputs=+-
  M_d_GG : Outport
  wires:
  Mux/1 -> M_d_GG/1
  Product2/1 -> Mux/2
  Product3/1 -> Mux/3
  Product1/1 -> Mux/1
  Matrix Multiply2/1 -> Demux3/1
  Subtract3/1 -> Product3/2
  Subtract1/1 -> Product1/2
  Subtract2/1 -> Product2/2
  Demux3/1 -> Product3/3, Product2/3
  "Ix, Iy, Iz"/1 -> Demux2/1
  Demux3/2 -> Product3/4, Product1/4
  Demux2/3 -> Subtract2/2, Subtract1/1
  Constant/1 -> Matrix Multiply2/2
  Demux2/2 -> Subtract3/1, Subtract1/2
  Demux3/3 -> Product2/4, Product1/3
  Demux2/1 -> Subtract3/2, Subtract2/1
  Gain/1 -> Product3/1, Product2/1, Product1/1
  A_bl/1 -> Matrix Multiply2/1
  R/1 -> Power/1
  Constant1/1 -> Power/2
  Divide/1 -> Gain/1
  Power/1 -> Divide/2
  Constant2/1 -> Divide/1
